simulink model "afe_abc_inv_psm_2mods"  (R2025a)
settings: Solver=ode1be  StartTime=0.0  StopTime=simlength  FixedStep=tc  MaxStep=tc
undefined symbols (not defined in the file): Ad_fht, Adrso, afe_pwm_phase_shift_mod1, afe_pwm_phase_shift_mod2, Amplitude_U, Amplitude_V, Amplitude_W, Aresd, b, Bresd, Cfht, Cresd, Crso, CTRPIFF_CLIP_RELEASE, dead_time_AFE, dead_time_INV, deepNEGeta, deepNEGxi, deepPOSxi, emf_fb_p, emf_fb_p_ccaller_1, emf_fb_p_ccaller_2, emf_p, emf_p_ccaller_1, emf_p_ccaller_2, enable_two_modules, end_time_LVRT, fPWM_AFE, fPWM_INV, g0_161Hz, g0_500Hz, g1_161Hz, g1_500Hz, i_grid_neg_eta_lim, i_grid_neg_eta_red_lim, i_grid_neg_xi_lim, i_grid_neg_xi_red_lim, i_grid_pos_eta_lim, i_grid_pos_eta_red_lim, ibez, id_lim, ieta_neg_ref_lim, ieta_pos_ref_lim, Igrid_phase_normalization_factor, inv_pwm_phase_shift_mod1, inv_pwm_phase_shift_mod2, iq_lim, ixi_pos_ref_lim, Jm, k_frt_ref, kg, ki_afe, ki_i, ki_rc_neg_grid, ki_rc_pos_grid, ki_vs, ki_w, kp_afe, kp_i, kp_rc_neg_grid ... (+64)
libraries: spsSampleandHoldLib x213, fl_lib x202, nesl_utility x126, simulink x22, cstblocks x18, threephase_inductor_lib x4, single_phase_transformer_lib x3, flexshaft_lib x1, pmsm_uvw_with_harmonics_lib x1
(part 13 of 18)

== system afe_abc_inv_psm_2mods/afe_abc_inv_psm_mod2/afe_control/voltage_sequence_avg/average_filter_ccaller/Moving Average Filter3 ==
  In2 : Inport
  In3 : Inport  Port=2
  Bus Selector : BusSelector  OutputSignals=ts,sshort,slong,pinput,cbpointer,cbsample,mavg_output
  C Caller : CCaller  FunctionName=mavgflt_process_simulink  PortSpecificationStruct="%)30     .    B H   8    (     @         %    \"     8    !     0         %  0 \"0    $    _    07)G3F%M90  4&]R=$YA;64 4V-O<&4     26YD97@     5'EP90      4VEZ90      27-';&]B86P   X    P    !@    @    $          4    (     0    ,    !         !   P!O=70 #@   #     &    \"     0         !0    @    !     P    $         $  # &]U=  .    .     8    (    !          %    \"     $    &     0         0   ...(+3251 chars)"  SampleTime=ts_afe
  Compare To Zero : simulink/Logic and Bit Operations/Compare To Zero  relop=>  OutDataTypeStr=boolean
  Constant : Constant  Value=11
  Constant5 : Constant  Value=ts_afe
  Data Type Conversion : DataTypeConversion  OutDataTypeStr=single  SaturateOnIntegerOverflow=off  RndMeth=Floor
  Data Type Conversion1 : DataTypeConversion  OutDataTypeStr=single  SaturateOnIntegerOverflow=off  RndMeth=Floor
  Data Type Conversion2 : DataTypeConversion  OutDataTypeStr=single  SaturateOnIntegerOverflow=off  RndMeth=Floor
  Data Type Conversion3 : DataTypeConversion  OutDataTypeStr=double  SaturateOnIntegerOverflow=off  RndMeth=Floor
  Data Type Conversion4 : DataTypeConversion  OutDataTypeStr=uint8  SaturateOnIntegerOverflow=off  RndMeth=Floor
  Data Type Conversion5 : DataTypeConversion  OutDataTypeStr=uint8  SaturateOnIntegerOverflow=off  RndMeth=Floor
  Enabled Subsystem : Subsystem  TreatAsAtomicUnit=on
  Reset Trigger : Subsystem
  Subsystem1 : Subsystem
      mask Display: disp('S/H afe mod 2');
  Subsystem2 : Subsystem
      mask Display: disp('S/H afe mod 2');
  Subsystem3 : Subsystem
      mask Display: disp('S/H afe mod 2');
  Subsystem4 : Subsystem
      mask Display: disp('S/H afe mod 2');
  Subsystem6 : Subsystem
      mask Display: disp('S/H afe mod 2');
  Terminator{,1..5} (6 alike) : Terminator
  Unit Delay{1..5} (5 alike) : UnitDelay  SampleTime=ts_afe  HasFrameUpgradeWarning=on
  xi : Outport
  wires:
  Subsystem4/1(Out) -> Unit Delay5/1
  Subsystem3/1(Out) -> Unit Delay4/1
  Subsystem2/1(Out) -> Unit Delay3/1
  Subsystem1/1(Out) -> Unit Delay2/1
  Subsystem6/1(Out) -> Unit Delay1/1
  Bus Selector/7 -> Data Type Conversion3/1  "<mavg_output>"
  Bus Selector/6 -> Terminator5/1  "<cbsample>"
  Constant/1 -> Data Type Conversion4/1
  Reset Trigger/1(Out1) -> Data Type Conversion5/1
  Data Type Conversion1/1 -> Subsystem1/1(In)
  Data Type Conversion2/1 -> Subsystem2/1(In)
  Data Type Conversion5/1 -> Subsystem3/1(In)
  Data Type Conversion/1 -> Subsystem6/1(In)
  Data Type Conversion4/1 -> Subsystem4/1(In)
  In2/1 -> Data Type Conversion/1  "input"
  C Caller/1 -> Bus Selector/1  "out"
  Bus Selector/1 -> Terminator/1  "<ts>"
  Bus Selector/2 -> Terminator3/1  "<sshort>"
  Bus Selector/3 -> Terminator4/1  "<slong>"
  Constant5/1 -> Data Type Conversion2/1  "d1"
  In3/1 -> Compare To Zero/1, Enabled Subsystem/1(In1)  "omega_grid"
  Compare To Zero/1 -> Enabled Subsystem/Enable
  Enabled Subsystem/1(Out1) -> Data Type Conversion1/1
  Data Type Conversion3/1 -> xi/1  "output"
  Bus Selector/4 -> Terminator1/1  "<pinput>"
  Bus Selector/5 -> Terminator2/1  "<cbpointer>"
  Unit Delay1/1 -> C Caller/1
  Unit Delay2/1 -> C Caller/2
  Unit Delay3/1 -> C Caller/3
  Unit Delay4/1 -> C Caller/4
  Unit Delay5/1 -> C Caller/5

== system afe_abc_inv_psm_2mods/afe_abc_inv_psm_mod2/afe_control/voltage_sequence_avg/average_filter_ccaller/Moving Average Filter4 ==
  In2 : Inport
  In3 : Inport  Port=2
  Bus Selector : BusSelector  OutputSignals=ts,sshort,slong,pinput,cbpointer,cbsample,mavg_output
  C Caller : CCaller  FunctionName=mavgflt_process_simulink  PortSpecificationStruct="%)30     .    B H   8    (     @         %    \"     8    !     0         %  0 \"0    $    _    07)G3F%M90  4&]R=$YA;64 4V-O<&4     26YD97@     5'EP90      4VEZ90      27-';&]B86P   X    P    !@    @    $          4    (     0    ,    !         !   P!O=70 #@   #     &    \"     0         !0    @    !     P    $         $  # &]U=  .    .     8    (    !          %    \"     $    &     0         0   ...(+3251 chars)"  SampleTime=ts_afe
  Compare To Zero : simulink/Logic and Bit Operations/Compare To Zero  relop=>  OutDataTypeStr=boolean
  Constant : Constant  Value=12
  Constant5 : Constant  Value=ts_afe
  Data Type Conversion : DataTypeConversion  OutDataTypeStr=single  SaturateOnIntegerOverflow=off  RndMeth=Floor
  Data Type Conversion1 : DataTypeConversion  OutDataTypeStr=single  SaturateOnIntegerOverflow=off  RndMeth=Floor
  Data Type Conversion2 : DataTypeConversion  OutDataTypeStr=single  SaturateOnIntegerOverflow=off  RndMeth=Floor
  Data Type Conversion3 : DataTypeConversion  OutDataTypeStr=double  SaturateOnIntegerOverflow=off  RndMeth=Floor
  Data Type Conversion4 : DataTypeConversion  OutDataTypeStr=uint8  SaturateOnIntegerOverflow=off  RndMeth=Floor
  Data Type Conversion5 : DataTypeConversion  OutDataTypeStr=uint8  SaturateOnIntegerOverflow=off  RndMeth=Floor
  Enabled Subsystem : Subsystem  TreatAsAtomicUnit=on
  Reset Trigger : Subsystem
  Subsystem1 : Subsystem
      mask Display: disp('S/H afe mod 2');
  Subsystem2 : Subsystem
      mask Display: disp('S/H afe mod 2');
  Subsystem3 : Subsystem
      mask Display: disp('S/H afe mod 2');
  Subsystem4 : Subsystem
      mask Display: disp('S/H afe mod 2');
  Subsystem6 : Subsystem
      mask Display: disp('S/H afe mod 2');
  Terminator{,1..5} (6 alike) : Terminator
  Unit Delay{1..5} (5 alike) : UnitDelay  SampleTime=ts_afe  HasFrameUpgradeWarning=on
  xi : Outport
  wires:
  Bus Selector/5 -> Terminator2/1  "<cbpointer>"
  Bus Selector/4 -> Terminator1/1  "<pinput>"
  Data Type Conversion3/1 -> xi/1  "output"
  Enabled Subsystem/1(Out1) -> Data Type Conversion1/1
  Compare To Zero/1 -> Enabled Subsystem/Enable
  In3/1 -> Enabled Subsystem/1(In1), Compare To Zero/1  "omega_grid"
  Constant5/1 -> Data Type Conversion2/1  "d1"
  Bus Selector/3 -> Terminator4/1  "<slong>"
  Bus Selector/2 -> Terminator3/1  "<sshort>"
  Bus Selector/1 -> Terminator/1  "<ts>"
  C Caller/1 -> Bus Selector/1  "out"
  In2/1 -> Data Type Conversion/1  "input"
  Data Type Conversion4/1 -> Subsystem4/1(In)
  Data Type Conversion/1 -> Subsystem6/1(In)
  Data Type Conversion5/1 -> Subsystem3/1(In)
  Data Type Conversion2/1 -> Subsystem2/1(In)
  Data Type Conversion1/1 -> Subsystem1/1(In)
  Reset Trigger/1(Out1) -> Data Type Conversion5/1
  Constant/1 -> Data Type Conversion4/1
  Bus Selector/6 -> Terminator5/1  "<cbsample>"
  Bus Selector/7 -> Data Type Conversion3/1  "<mavg_output>"
  Subsystem6/1(Out) -> Unit Delay1/1
  Subsystem1/1(Out) -> Unit Delay2/1
  Subsystem2/1(Out) -> Unit Delay3/1
  Subsystem3/1(Out) -> Unit Delay4/1
  Subsystem4/1(Out) -> Unit Delay5/1
  Unit Delay1/1 -> C Caller/1
  Unit Delay2/1 -> C Caller/2
  Unit Delay3/1 -> C Caller/3
  Unit Delay4/1 -> C Caller/4
  Unit Delay5/1 -> C Caller/5

== system afe_abc_inv_psm_2mods/afe_abc_inv_psm_mod2/afe_control/voltage_sequence_avg/average_filter_simulink/moving_avarage_1 ==
  in : Inport
  Gain : Gain  Gain=n1-1
  Gain1 : Gain  Gain=1/n1
  Sum : Sum  Inputs=|++
  Unit Delay : UnitDelay  SampleTime=ts_afe  HasFrameUpgradeWarning=on
  out : Outport  VectorParamsAs1DForOutWhenUnconnected=off
  wires:
  Gain/1 -> Sum/2
  Gain1/1 -> out/1, Unit Delay/1
  in/1 -> Sum/1
  Unit Delay/1 -> Gain/1
  Sum/1 -> Gain1/1

== system afe_abc_inv_psm_2mods/afe_abc_inv_psm_mod2/afe_control/voltage_sequence_avg/average_filter_simulink/moving_avarage_2 ==
  in : Inport
  Gain : Gain  Gain=n1-1
  Gain1 : Gain  Gain=1/n1
  Sum : Sum  Inputs=|++
  Unit Delay : UnitDelay  SampleTime=ts_afe  HasFrameUpgradeWarning=on
  out : Outport  VectorParamsAs1DForOutWhenUnconnected=off
  wires:
  Sum/1 -> Gain1/1
  Unit Delay/1 -> Gain/1
  in/1 -> Sum/1
  Gain1/1 -> Unit Delay/1, out/1
  Gain/1 -> Sum/2

== system afe_abc_inv_psm_2mods/afe_abc_inv_psm_mod2/afe_control/voltage_sequence_avg/average_filter_simulink/moving_avarage_3 ==
  in : Inport
  Gain : Gain  Gain=n1-1
  Gain1 : Gain  Gain=1/n1
  Sum : Sum  Inputs=|++
  Unit Delay : UnitDelay  SampleTime=ts_afe  HasFrameUpgradeWarning=on
  out : Outport  VectorParamsAs1DForOutWhenUnconnected=off
  wires:
  Gain/1 -> Sum/2
  Gain1/1 -> out/1, Unit Delay/1
  in/1 -> Sum/1
  Unit Delay/1 -> Gain/1
  Sum/1 -> Gain1/1

== system afe_abc_inv_psm_2mods/afe_abc_inv_psm_mod2/afe_control/voltage_sequence_avg/average_filter_simulink/moving_avarage_4 ==
  in : Inport
  Gain : Gain  Gain=n1-1
  Gain1 : Gain  Gain=1/n1
  Sum : Sum  Inputs=|++
  Unit Delay : UnitDelay  SampleTime=ts_afe  HasFrameUpgradeWarning=on
  out : Outport  VectorParamsAs1DForOutWhenUnconnected=off
  wires:
  Sum/1 -> Gain1/1
  Unit Delay/1 -> Gain/1
  in/1 -> Sum/1
  Gain1/1 -> Unit Delay/1, out/1
  Gain/1 -> Sum/2

== system afe_abc_inv_psm_2mods/afe_abc_inv_psm_mod2/inverter/inverter/sv_pwm/Subsystem1 ==
  In : Inport
  Sample and Hold : spsSampleandHoldLib/Sample and Hold  ic=0  Ts=0
  Out : Outport
  wires:
  In/1 -> Sample and Hold/1
  [TRGO_inv_module_1] -> Sample and Hold/2
  Sample and Hold/1 -> Out/1

== system afe_abc_inv_psm_2mods/afe_abc_inv_psm_mod2/inverter/inverter/sv_pwm/Subsystem2 ==
  In : Inport
  Sample and Hold : spsSampleandHoldLib/Sample and Hold  ic=0  Ts=0
  Out : Outport
  wires:
  Sample and Hold/1 -> Out/1
  [TRGO_inv_module_1] -> Sample and Hold/2
  In/1 -> Sample and Hold/1

== system afe_abc_inv_psm_2mods/afe_abc_inv_psm_mod2/inverter/inverter/sv_pwm/Subsystem3 ==
  In : Inport
  Sample and Hold : spsSampleandHoldLib/Sample and Hold  ic=0  Ts=0
  Out : Outport
  wires:
  In/1 -> Sample and Hold/1
  [TRGO_inv_module_1] -> Sample and Hold/2
  Sample and Hold/1 -> Out/1

== system afe_abc_inv_psm_2mods/afe_abc_inv_psm_mod2/inverter/inverter/sv_pwm/Subsystem4 ==
  In : Inport
  Sample and Hold : spsSampleandHoldLib/Sample and Hold  ic=0  Ts=0
  Out : Outport
  wires:
  Sample and Hold/1 -> Out/1
  [TRGO_inv_module_1] -> Sample and Hold/2
  In/1 -> Sample and Hold/1

== system afe_abc_inv_psm_2mods/afe_abc_inv_psm_mod2/inverter/inverter/sv_pwm/modulator1 ==
  u : Inport
  v : Inport  Port=2
  w : Inport  Port=3
  phase : Inport  Port=4
  Bus Creator3 : BusCreator  Inputs=6
  PWM generator 1 : Subsystem  mask{f=fPWM_INV, m_up=0.98, m_low=0.02, dead_time=dead_time_INV, pos_cmd_gate=15, neg_cmd_gate=-10, polarity=1}
      mask prompts: f "Frequency (Hz)"; m_up "Max Input Modulation Value"; m_low "Min Input Modulation Value"; dead_time "Dead Time (s)"; pos_cmd_gate "Positive Gate Voltage (V)"; neg_cmd_gate "Negative Gate Voltage (V)"; polarity "Polarity (pu)"
  PWM generator 2 : Subsystem  mask{f=fPWM_INV, m_up=0.98, m_low=0.02, dead_time=dead_time_INV, pos_cmd_gate=15, neg_cmd_gate=-10, polarity=1}
      mask prompts: f "Frequency (Hz)"; m_up "Max Input Modulation Value"; m_low "Min Input Modulation Value"; dead_time "Dead Time (s)"; pos_cmd_gate "Positive Gate Voltage (V)"; neg_cmd_gate "Negative Gate Voltage (V)"; polarity "Polarity (pu)"
  PWM generator 3 : Subsystem  mask{f=fPWM_INV, m_up=0.98, m_low=0.02, dead_time=dead_time_INV, pos_cmd_gate=15, neg_cmd_gate=-10, polarity=1}
      mask prompts: f "Frequency (Hz)"; m_up "Max Input Modulation Value"; m_low "Min Input Modulation Value"; dead_time "Dead Time (s)"; pos_cmd_gate "Positive Gate Voltage (V)"; neg_cmd_gate "Negative Gate Voltage (V)"; polarity "Polarity (pu)"
  cmd_gates : Outport
  wires:
  Bus Creator3/1 -> cmd_gates/1
  PWM generator 1/1(m1) -> Bus Creator3/1  "pwm_inverter_phase_u_top"
  PWM generator 3/2(m2) -> Bus Creator3/6  "pwm_inverter_phase_w_bottom"
  PWM generator 2/2(m2) -> Bus Creator3/4  "pwm_inverter_phase_v_bottom"
  PWM generator 2/1(m1) -> Bus Creator3/3  "pwm_inverter_phase_v_top"
  PWM generator 3/1(m1) -> Bus Creator3/5  "pwm_inverter_phase_w_top"
  PWM generator 1/2(m2) -> Bus Creator3/2  "pwm_inverter_phase_u_bottom"
  phase/1 -> PWM generator 1/2(phase), PWM generator 2/2(phase), PWM generator 3/2(phase)
  v/1 -> PWM generator 2/1(m_index)
  w/1 -> PWM generator 3/1(m_index)
  u/1 -> PWM generator 1/1(m_index)

== system afe_abc_inv_psm_2mods/afe_abc_inv_psm_mod2/inverter_control/current_ctrl/bemf_observer/bemf_observer ==
  ialpha_pu : Inport
  ibeta_pu : Inport  Port=2
  ualpha_pu : Inport  Port=3
  ubeta_pu : Inport  Port=4
  Gain : Gain  Gain=psi_m_norm
  Gain1 : Gain  Gain=psi_m_norm
  Trigonometric Function : Trigonometry  Operator=cos
  Trigonometric Function1 : Trigonometry
  double_integrator_observer : Subsystem
  psi_alpha_hat : Subsystem
  psi_beta_hat : Subsystem
  theta_bemf_hat : Subsystem
  omega_pu : Outport
  theta_hat : Outport  Port=2
  tag scope: psi_r_alpha_hat_mod2=global, psi_r_alpha_pu_hat_mod2=global, psi_r_beta_hat_mod2=global, psi_r_beta_pu_hat_mod2=global, psi_r_m_alpha_mod2=global, psi_r_m_beta_mod2=global, theta_bemf_hat_mod2=global
  wires:
  [psi_r_beta_hat_mod2] -> [psi_r_beta_pu_hat_mod2]
  [psi_r_alpha_hat_mod2] -> [psi_r_alpha_pu_hat_mod2]
  double_integrator_observer/2(theta_hat) -> theta_hat/1
  double_integrator_observer/1(omega_pu_hat) -> omega_pu/1
  [theta_bemf_hat_mod2] -> double_integrator_observer/1(theta)
  theta_bemf_hat/1(theta_emf_hat) -> [theta_bemf_hat_mod2]
  Gain1/1 -> [psi_r_m_beta_mod2]
  Gain/1 -> [psi_r_m_alpha_mod2]
  [theta_hat_mod2] -> Trigonometric Function1/1, Trigonometric Function/1
  ubeta_pu/1 -> psi_beta_hat/1(ubeta)
  ualpha_pu/1 -> psi_alpha_hat/1(ualpha)
  [psi_r_beta_hat_mod2] -> theta_bemf_hat/2(psi_r_beta_hat)
  [psi_r_alpha_hat_mod2] -> theta_bemf_hat/1(psi_r_alpha_hat)
  psi_beta_hat/2(psi_r_beta_hat) -> [psi_r_beta_hat_mod2]
  psi_alpha_hat/2(psi_r_alpha_hat) -> [psi_r_alpha_hat_mod2]
  ibeta_pu/1 -> psi_beta_hat/2(ibeta)
  ialpha_pu/1 -> psi_alpha_hat/2(ialpha)
  Trigonometric Function1/1 -> Gain1/1
  Trigonometric Function/1 -> Gain/1

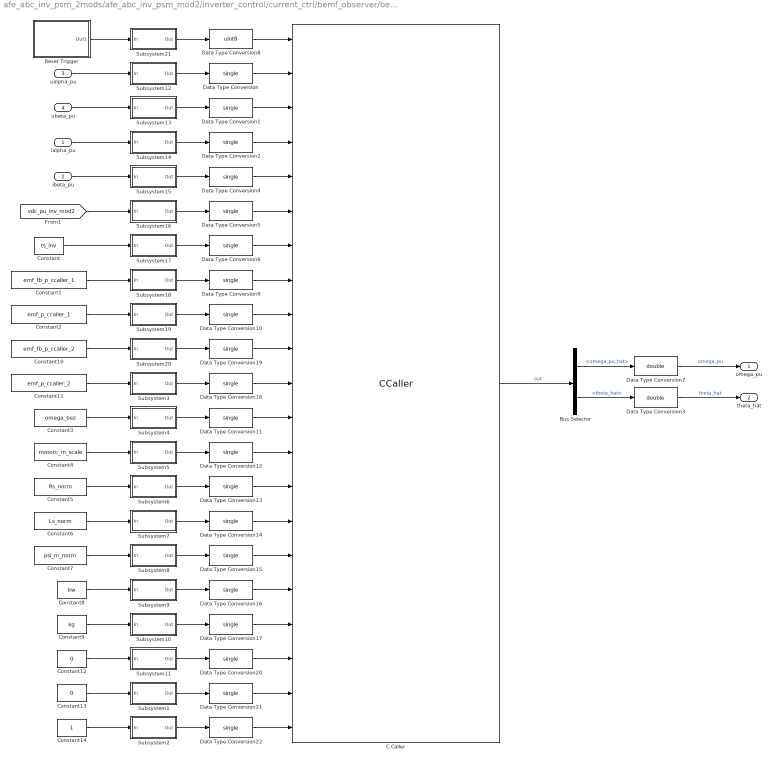
== system afe_abc_inv_psm_2mods/afe_abc_inv_psm_mod2/inverter_control/current_ctrl/bemf_observer/bemf_observer_ccaller ==
  ialpha_pu : Inport
  ibeta_pu : Inport  Port=2
  ualpha_pu : Inport  Port=3
  ubeta_pu : Inport  Port=4
  Bus Selector : BusSelector  OutputSignals=omega_pu_hat,theta_hat
  C Caller : CCaller  FunctionName=bemf_obsv_process_simulink  PortSpecificationStruct="%)30     .    N\"8   8    (     @         %    \"    !8    !     0         %  0 \"0    $    _    07)G3F%M90  4&]R=$YA;64 4V-O<&4     26YD97@     5'EP90      4VEZ90      27-';&]B86P   X    P    !@    @    $          4    (     0    ,    !         !   P!O=70 #@   #     &    \"     0         !0    @    !     P    $         $  # &]U=  .    .     8    (    !          %    \"     $    &     0         0  ...(+12985 chars)"  SampleTime=ts_inv
  Constant : Constant  Value=ts_inv
  Constant1 : Constant  Value=emf_fb_p_ccaller_1
  Constant10 : Constant  Value=emf_fb_p_ccaller_2
  Constant11 : Constant  Value=emf_p_ccaller_2
  Constant12 : Constant  Value=0
  Constant13 : Constant  Value=0
  Constant14 : Constant
  Constant2 : Constant  Value=emf_p_ccaller_1
  Constant3 : Constant  Value=omega_bez
  Constant4 : Constant  Value=motorc_m_scale
  Constant5 : Constant  Value=Rs_norm
  Constant6 : Constant  Value=Ls_norm
  Constant7 : Constant  Value=psi_m_norm
  Constant8 : Constant  Value=kw
  Constant9 : Constant  Value=kg
  Data Type Conversion{,1..2,4..6,9..22} (20 alike) : DataTypeConversion  OutDataTypeStr=single  SaturateOnIntegerOverflow=off  RndMeth=Floor
  Data Type Conversion3 : DataTypeConversion  OutDataTypeStr=double  SaturateOnIntegerOverflow=off  RndMeth=Floor
  Data Type Conversion7 : DataTypeConversion  OutDataTypeStr=double  SaturateOnIntegerOverflow=off  RndMeth=Floor
  Data Type Conversion8 : DataTypeConversion  OutDataTypeStr=uint8  SaturateOnIntegerOverflow=off  RndMeth=Floor
  Reset Trigger : Subsystem
  Subsystem1 : Subsystem
      mask Display: disp('S/H inv mod 2');
  Subsystem10 : Subsystem
      mask Display: disp('S/H inv mod 2');
  Subsystem11 : Subsystem
      mask Display: disp('S/H inv mod 2');
  Subsystem12 : Subsystem
      mask Display: disp('S/H inv mod 2');
  Subsystem13 : Subsystem
      mask Display: disp('S/H inv mod 2');
  Subsystem14 : Subsystem
      mask Display: disp('S/H inv mod 2');
  Subsystem15 : Subsystem
      mask Display: disp('S/H inv mod 2');
  Subsystem16 : Subsystem
      mask Display: disp('S/H inv mod 2');
  Subsystem17 : Subsystem
      mask Display: disp('S/H inv mod 2');
  Subsystem18 : Subsystem
      mask Display: disp('S/H inv mod 2');
  Subsystem19 : Subsystem
      mask Display: disp('S/H inv mod 2');
  Subsystem2 : Subsystem
      mask Display: disp('S/H inv mod 2');
  Subsystem20 : Subsystem
      mask Display: disp('S/H inv mod 2');
  Subsystem21 : Subsystem
      mask Display: disp('S/H inv mod 2');
  Subsystem3 : Subsystem
      mask Display: disp('S/H inv mod 2');
  Subsystem4 : Subsystem
      mask Display: disp('S/H inv mod 2');
  Subsystem5 : Subsystem
      mask Display: disp('S/H inv mod 2');
  Subsystem6 : Subsystem
      mask Display: disp('S/H inv mod 2');
  Subsystem7 : Subsystem
      mask Display: disp('S/H inv mod 2');
  Subsystem8 : Subsystem
      mask Display: disp('S/H inv mod 2');
  Subsystem9 : Subsystem
      mask Display: disp('S/H inv mod 2');
  omega_pu : Outport
  theta_hat : Outport  Port=2
  wires:
  Subsystem21/1(Out) -> Data Type Conversion8/1
  Subsystem12/1(Out) -> Data Type Conversion/1
  Subsystem13/1(Out) -> Data Type Conversion1/1
  Subsystem14/1(Out) -> Data Type Conversion2/1
  Subsystem15/1(Out) -> Data Type Conversion4/1
  Subsystem16/1(Out) -> Data Type Conversion5/1
  Subsystem17/1(Out) -> Data Type Conversion6/1
  Subsystem18/1(Out) -> Data Type Conversion9/1
  Subsystem19/1(Out) -> Data Type Conversion10/1
  Subsystem20/1(Out) -> Data Type Conversion19/1
  Subsystem3/1(Out) -> Data Type Conversion18/1
  Subsystem4/1(Out) -> Data Type Conversion11/1
  Subsystem5/1(Out) -> Data Type Conversion12/1
  Subsystem6/1(Out) -> Data Type Conversion13/1
  Subsystem7/1(Out) -> Data Type Conversion14/1
  Subsystem8/1(Out) -> Data Type Conversion15/1
  Subsystem9/1(Out) -> Data Type Conversion16/1
  Subsystem10/1(Out) -> Data Type Conversion17/1
  Subsystem11/1(Out) -> Data Type Conversion20/1
  Subsystem1/1(Out) -> Data Type Conversion21/1
  Subsystem2/1(Out) -> Data Type Conversion22/1
  Data Type Conversion22/1 -> C Caller/21
  Constant14/1 -> Subsystem2/1(In)
  Data Type Conversion21/1 -> C Caller/20
  Constant13/1 -> Subsystem1/1(In)
  Constant12/1 -> Subsystem11/1(In)
  Data Type Conversion20/1 -> C Caller/19
  Data Type Conversion17/1 -> C Caller/18
  Data Type Conversion16/1 -> C Caller/17
  Data Type Conversion15/1 -> C Caller/16
  Data Type Conversion14/1 -> C Caller/15
  Data Type Conversion13/1 -> C Caller/14
  Data Type Conversion12/1 -> C Caller/13
  Data Type Conversion11/1 -> C Caller/12
  Data Type Conversion18/1 -> C Caller/11
  Data Type Conversion19/1 -> C Caller/10
  Constant10/1 -> Subsystem20/1(In)
  Constant11/1 -> Subsystem3/1(In)
  Constant9/1 -> Subsystem10/1(In)
  Constant8/1 -> Subsystem9/1(In)
  Constant7/1 -> Subsystem8/1(In)
  Constant6/1 -> Subsystem7/1(In)
  Constant5/1 -> Subsystem6/1(In)
  Constant4/1 -> Subsystem5/1(In)
  Constant3/1 -> Subsystem4/1(In)
  Constant2/1 -> Subsystem19/1(In)
  Data Type Conversion10/1 -> C Caller/9
  Data Type Conversion9/1 -> C Caller/8
  Constant1/1 -> Subsystem18/1(In)
  Data Type Conversion8/1 -> C Caller/1
  Reset Trigger/1(Out1) -> Subsystem21/1(In)
  Data Type Conversion3/1 -> theta_hat/1  "theta_hat"
  Data Type Conversion7/1 -> omega_pu/1  "omega_pu"
  Bus Selector/1 -> Data Type Conversion7/1  "<omega_pu_hat>"
  Bus Selector/2 -> Data Type Conversion3/1  "<theta_hat>"
  [vdc_pu_inv_mod2] -> Subsystem16/1(In)
  ibeta_pu/1 -> Subsystem15/1(In)
  ialpha_pu/1 -> Subsystem14/1(In)
  ubeta_pu/1 -> Subsystem13/1(In)
  ualpha_pu/1 -> Subsystem12/1(In)
  Constant/1 -> Subsystem17/1(In)
  Data Type Conversion6/1 -> C Caller/7
  Data Type Conversion2/1 -> C Caller/4
  Data Type Conversion4/1 -> C Caller/5
  Data Type Conversion1/1 -> C Caller/3
  C Caller/1 -> Bus Selector/1  "out"
  Data Type Conversion/1 -> C Caller/2
  Data Type Conversion5/1 -> C Caller/6

== system afe_abc_inv_psm_2mods/afe_abc_inv_psm_mod2/inverter_control/current_ctrl/bemf_observer/phase_fault ==
  double_integrator_observer : Subsystem
  phase_fault : Subsystem
  omega_pu_encoder : Outport
  theta_hat_encoder : Outport  Port=2
  wires:
  double_integrator_observer/1(omega_pu_hat) -> omega_pu_encoder/1  "omega_pu_encoder"
  phase_fault/1(theta) -> double_integrator_observer/1(theta)
  double_integrator_observer/2(theta_hat) -> theta_hat_encoder/1  "theta_hat_encoder"
  [theta_elec_psm] -> phase_fault/1(theta_pmsm)  "theta_pmsm"

== system afe_abc_inv_psm_2mods/afe_abc_inv_psm_mod2/inverter_control/current_ctrl/current_ctrl/MTPA ==
  iq_ref : Inport
  Gain1 : Gain  Gain=1/(Ld_norm - Lq_norm)/2
  Gain2 : Gain  Gain=1/(Ld_norm - Lq_norm)/2
  Gain3 : Gain  Gain=-1
  Math Function1 : Math  Operator=magnitude^2  SignedPower=on
  Math Function4 : Math  Operator=magnitude^2  SignedPower=on
  Sqrt : Sqrt
  Sum : Sum  Inputs=|++
  Sum1 : Sum  Inputs=|-+
  id_ref_pu < x < 0 : Saturate  UpperLimit=0  LowerLimit=-id_lim
  Id_ref_mtpa : Outport  VectorParamsAs1DForOutWhenUnconnected=off
  wires:
  Gain3/1 -> id_ref_pu < x < 0/1
  [omega_hat_pu_mod2] -> Gain2/1, Gain1/1
  Gain2/1 -> Sum1/1
  iq_ref/1 -> Math Function1/1
  Sqrt/1 -> Sum1/2
  Sum/1 -> Sqrt/1
  Gain1/1 -> Math Function4/1
  Math Function1/1 -> Sum/2
  Math Function4/1 -> Sum/1
  id_ref_pu < x < 0/1 -> Id_ref_mtpa/1
  Sum1/1 -> Gain3/1

== system afe_abc_inv_psm_2mods/afe_abc_inv_psm_mod2/inverter_control/current_ctrl/current_ctrl/dq_pi_with_vector_antiwindup ==
  id_ref : Inport
  id : Inport  Port=2
  iq_ref : Inport  Port=3
  iq : Inport  Port=4
  Variant Source : VariantSource  VariantControls={use_current_controller_from_simulink_module_2 == 1, use_current_controller_from_ccaller_module_2 == 1}
  Variant Source1 : VariantSource  VariantControls={use_current_controller_from_simulink_module_2 == 1, use_current_controller_from_ccaller_module_2 == 1}
  dq_vector_pi : Subsystem
  dq_vector_pi_ccaller : Subsystem
  simulink/Ccaller VectorPI : Scope  NumInputPorts=2
      settings: SampleTime=tc  ActiveDisplayYMinimum=-0.1324  ActiveDisplayYMaximum=0.52503
  ctrl_d_u : Outport
  ctrl_q_u : Outport  Port=2
  wires:
  Variant Source1/1 -> ctrl_q_u/1, simulink/Ccaller VectorPI/2
  Variant Source/1 -> simulink/Ccaller VectorPI/1, ctrl_d_u/1
  dq_vector_pi_ccaller/1(ud_ctrl_out) -> Variant Source/2
  dq_vector_pi/2(mq_sat) -> Variant Source1/1
  dq_vector_pi_ccaller/2(uq_ctrl_out) -> Variant Source1/2
  dq_vector_pi/1(md_sat) -> Variant Source/1
  iq_ref/1 -> dq_vector_pi_ccaller/4(iq_ref), dq_vector_pi/4(iq_ref)  "iq_ref"
  iq/1 -> dq_vector_pi/3(iq), dq_vector_pi_ccaller/3(iq)  "iq"
  id_ref/1 -> dq_vector_pi/2(id_ref), dq_vector_pi_ccaller/2(id_ref)  "id_ref"
  id/1 -> dq_vector_pi/1(id), dq_vector_pi_ccaller/1(id)  "id"

== system afe_abc_inv_psm_2mods/afe_abc_inv_psm_mod2/inverter_control/current_ctrl/current_ctrl/id_ref ==
  id_mtpa : Inport
  Constant : Constant  Value=0
  Variant Source : VariantSource  VariantControls={use_mtpa == 1, use_mtpa == 0}
  id_ref : Outport
  wires:
  Constant/1 -> Variant Source/2
  id_mtpa/1 -> Variant Source/1
  Variant Source/1 -> id_ref/1

== system afe_abc_inv_psm_2mods/afe_abc_inv_psm_mod2/inverter_control/current_ctrl/sample_hold_normalization/Subsystem1 ==
  In : Inport
  Sample and Hold : spsSampleandHoldLib/Sample and Hold  ic=0  Ts=0
  Out : Outport
  wires:
  Sample and Hold/1 -> Out/1
  [TRGO_inv_module_2] -> Sample and Hold/2
  In/1 -> Sample and Hold/1

== system afe_abc_inv_psm_2mods/afe_abc_inv_psm_mod2/inverter_control/current_ctrl/sample_hold_normalization/Subsystem2 ==
  In : Inport
  Sample and Hold : spsSampleandHoldLib/Sample and Hold  ic=0  Ts=0
  Out : Outport
  wires:
  In/1 -> Sample and Hold/1
  [TRGO_inv_module_2] -> Sample and Hold/2
  Sample and Hold/1 -> Out/1

== system afe_abc_inv_psm_2mods/afe_abc_inv_psm_mod2/inverter_control/current_ctrl/sample_hold_normalization/Subsystem5 ==
  In : Inport
  Sample and Hold : spsSampleandHoldLib/Sample and Hold  ic=0  Ts=0
  Out : Outport
  wires:
  Sample and Hold/1 -> Out/1
  [TRGO_inv_module_2] -> Sample and Hold/2
  In/1 -> Sample and Hold/1

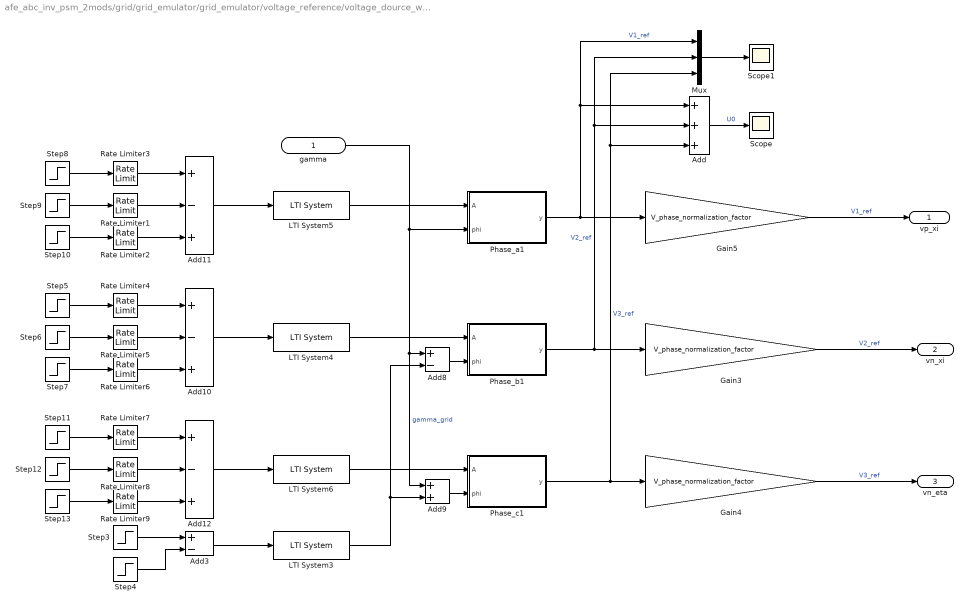
== system afe_abc_inv_psm_2mods/grid/grid_emulator/grid_emulator/voltage_reference/voltage_dource_with_frt ==
  gamma : Inport
  Add : Sum  Inputs=+++
  Add10 : Sum  Inputs=+-+
  Add11 : Sum  Inputs=+-+
  Add12 : Sum  Inputs=+-+
  Add3 : Sum  Inputs=+-
  Add8 : Sum  Inputs=+-
  Add9 : Sum
  Gain3 : Gain  Gain=V_phase_normalization_factor
  Gain4 : Gain  Gain=V_phase_normalization_factor
  Gain5 : Gain  Gain=V_phase_normalization_factor
  LTI System{3..6} (4 alike) : cstblocks/LTI System  sys=LVRT_flt_ss_c  IC=[0]  PadeOrder=0
  Mux : Mux  Inputs=3
  Phase_a1 : MATLAB Function  TreatAsAtomicUnit=on
  Phase_b1 : MATLAB Function  TreatAsAtomicUnit=on
  Phase_c1 : MATLAB Function  TreatAsAtomicUnit=on
  Rate Limiter{1..9} (9 alike) : RateLimiter  RisingSlewLimit=Vemu_ref_norm/t_ramp  FallingSlewLimit=-Vemu_ref_norm/t_ramp  SampleTimeMode=inherited
  Scope : Scope
      settings: ActiveDisplayYMinimum=-1E-15  ActiveDisplayYMaximum=8E-16
  Scope1 : Scope
      settings: ActiveDisplayYMinimum=-1.25511  ActiveDisplayYMaximum=1.25511
  Step10 : Step  Time=end_time_LVRT  After=Vemu_ref_norm*(1-Amplitude_U)  SampleTime=0
  Step11 : Step  Time=0  After=Vemu_ref_norm  SampleTime=0
  Step12 : Step  Time=start_time_LVRT  After=Vemu_ref_norm*(1-Amplitude_W)  SampleTime=0
  Step13 : Step  Time=end_time_LVRT  After=Vemu_ref_norm*(1-Amplitude_W)  SampleTime=0
  Step3 : Step  Time=start_time_LVRT  After=Phase_shift  SampleTime=0
  Step4 : Step  Time=end_time_LVRT  After=Phase_shift  SampleTime=0
  Step5 : Step  Time=0  After=Vemu_ref_norm  SampleTime=0
  Step6 : Step  Time=start_time_LVRT  After=Vemu_ref_norm*(1-Amplitude_V)  SampleTime=0
  Step7 : Step  Time=end_time_LVRT  After=Vemu_ref_norm*(1-Amplitude_V)  SampleTime=0
  Step8 : Step  Time=0  After=Vemu_ref_norm  SampleTime=0
  Step9 : Step  Time=start_time_LVRT  After=Vemu_ref_norm*(1-Amplitude_U)  SampleTime=0
  vp_xi : Outport  VectorParamsAs1DForOutWhenUnconnected=off
  vn_xi : Outport  Port=2  VectorParamsAs1DForOutWhenUnconnected=off
  vn_eta : Outport  Port=3  VectorParamsAs1DForOutWhenUnconnected=off
  wires:
  Phase_c1/1(y) -> Mux/3, Add/3, Gain4/1  "V3_ref"
  LTI System6/1 -> Phase_c1/1(A)
  gamma/1 -> Add9/1, Add8/1, Phase_a1/2(phi)  "gamma_grid"
  Add9/1 -> Phase_c1/2(phi)
  Add8/1 -> Phase_b1/2(phi)
  Phase_b1/1(y) -> Mux/2, Add/2, Gain3/1  "V2_ref"
  Phase_a1/1(y) -> Mux/1, Add/1, Gain5/1  "V1_ref"
  LTI System4/1 -> Phase_b1/1(A)
  Step5/1 -> Rate Limiter4/1
  Step6/1 -> Rate Limiter5/1
  Step7/1 -> Rate Limiter6/1
  Add10/1 -> LTI System4/1
  Step8/1 -> Rate Limiter3/1
  Add11/1 -> LTI System5/1
  Step9/1 -> Rate Limiter1/1
  Step10/1 -> Rate Limiter2/1
  LTI System5/1 -> Phase_a1/1(A)
  Add12/1 -> LTI System6/1
  Rate Limiter3/1 -> Add11/1
  Rate Limiter1/1 -> Add11/2
  Rate Limiter2/1 -> Add11/3
  Rate Limiter4/1 -> Add10/1
  Rate Limiter5/1 -> Add10/2
  Rate Limiter6/1 -> Add10/3
  Step12/1 -> Rate Limiter8/1
  Rate Limiter8/1 -> Add12/2
  Step13/1 -> Rate Limiter9/1
  Rate Limiter9/1 -> Add12/3
  Step11/1 -> Rate Limiter7/1
  Rate Limiter7/1 -> Add12/1
  Gain5/1 -> vp_xi/1  "V1_ref"
  Gain3/1 -> vn_xi/1  "V2_ref"
  Gain4/1 -> vn_eta/1  "V3_ref"
  Add3/1 -> LTI System3/1
  Step3/1 -> Add3/1
  Step4/1 -> Add3/2
  LTI System3/1 -> Add9/2, Add8/2
  Add/1 -> Scope/1  "U0"
  Mux/1 -> Scope1/1

== system afe_abc_inv_psm_2mods/afe_abc_inv_psm_mod1/afe_control/current_sequence_avg/average_filter_ccaller/Moving Average Filter5/Enabled Subsystem ==
  In1 : Inport
  Enable : EnablePort
  Constant2 : Constant
  Divide : Product  Inputs=*/
  Gain1 : Gain  Gain=1/(2*pi)
  Gain9 : Gain  Gain=mavarage_filter_frequency_base_order
  Out1 : Outport
  wires:
  Constant2/1 -> Divide/1
  In1/1 -> Gain1/1  "Omega_el"
  Gain9/1 -> Divide/2
  Divide/1 -> Out1/1  "period"
  Gain1/1 -> Gain9/1

== system afe_abc_inv_psm_2mods/afe_abc_inv_psm_mod1/afe_control/current_sequence_avg/average_filter_ccaller/Moving Average Filter5/Reset Trigger ==
  Constant1 : Constant  Value=simlength
  Constant3 : Constant  Value=0
  Constant4 : Constant
  Mod : Math  Operator=mod
  Switch : Switch  Criteria=u2 ~= 0  SaturateOnIntegerOverflow=off  InputSameDT=off
  Out1 : Outport
  wires:
  [TRGO_afe_module_1] -> Mod/1
  Constant3/1 -> Switch/1
  Constant4/1 -> Switch/3
  Mod/1 -> Switch/2
  Switch/1 -> Out1/1  "Reset"
  Constant1/1 -> Mod/2

== system afe_abc_inv_psm_2mods/afe_abc_inv_psm_mod1/afe_control/current_sequence_avg/average_filter_ccaller/Moving Average Filter5/Subsystem1 ==
  In : Inport
  Sample and Hold : spsSampleandHoldLib/Sample and Hold  ic=0  Ts=0
  Out : Outport
  wires:
  In/1 -> Sample and Hold/1
  [TRGO_afe_module_1] -> Sample and Hold/2
  Sample and Hold/1 -> Out/1

== system afe_abc_inv_psm_2mods/afe_abc_inv_psm_mod1/afe_control/current_sequence_avg/average_filter_ccaller/Moving Average Filter5/Subsystem2 ==
  In : Inport
  Sample and Hold : spsSampleandHoldLib/Sample and Hold  ic=0  Ts=0
  Out : Outport
  wires:
  Sample and Hold/1 -> Out/1
  [TRGO_afe_module_1] -> Sample and Hold/2
  In/1 -> Sample and Hold/1
